simulink model "Joystick_HIL"  (R2025b)
settings: Solver=FixedStepDiscrete  StartTime=0.0  StopTime=inf  RelTol=1e-3
undefined symbols (not defined in the file): battery_voltage, force_table, pwm_list, voltage_list
libraries: ros2lib x3
settings Model: Creator=vulcangrip  LastModifiedBy=vulcangrip
settings OptimizationCC: DefaultParameterBehavior=Inlined  EnhancedBackFolding=on  PassReuseOutputArgsAs=Individual arguments  ZeroExternalMemoryAtStartup=off  ZeroInternalMemoryAtStartup=off  OptimizeBlockOrder=speed  DifferentSizesBufferReuse=on  OptimizationCustomize=off  EfficientTunableParamExpr=on
settings DebuggingCC: ParameterTunabilityLossMsg=error
settings SFSimCC: MATLABDynamicMemAlloc=off  SimTargetLang=C++  SimDLTargetLibrary=mkl-dnn
settings RTWCC: SystemTargetFile=ert.tlc  GenCodeOnly=on  TemplateMakefile=ert_default_tmf  Toolchain=CMake  TargetLang=C++  Description=Embedded Coder
settings CodeAppCC: ForceParamTrailComments=on  IgnoreCustomStorageClasses=off  OperatorAnnotations=on  SimulinkDataObjDesc=on  SFDataObjDesc=on  InsertBlockDesc=on
settings ERTTargetCC: RootIOFormat=Structure reference  ERTCustomFileTemplate=example_file_process.tlc  TargetLangStandard=C++11 (ISO)  GenerateSampleERTMain=on  CodeInterfacePackaging=C++ class  SubcomponentCodeInterfacePackaging=C++ class
settings ConfigComp: CovScope=ReferencedModels

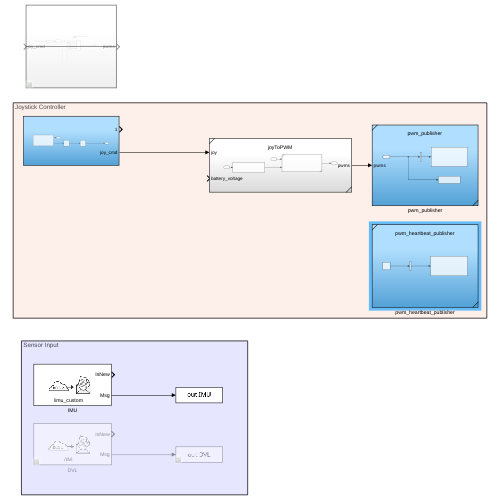
[thumbnail: Simulink's stored preview of the top-level diagram]
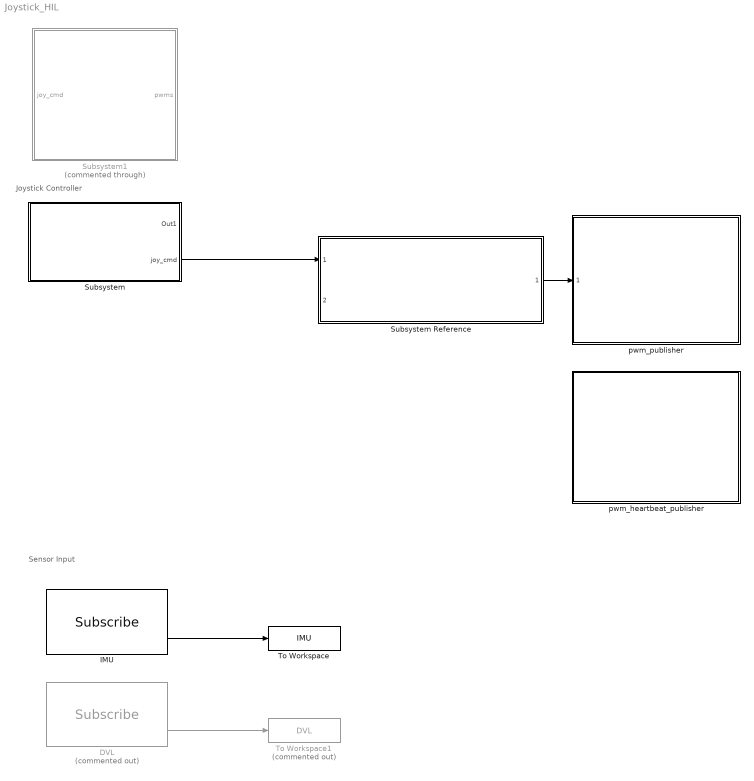
== system Joystick_HIL ==
  note: Joystick Controller
  note: Sensor Input
  DVL : ros2lib/Subscribe  Commented=on  topicSource=Specify your own  topic=/dvl  messageType=custom_interfaces/Position  sampleTime=-1  QOSHistory=Keep last  QOSDepth=10  QOSReliability=Reliable  QOSDurability=Volatile  QOSDeadline=Inf  QOSLifespan=Inf  QOSLiveliness=Automatic  QOSLeaseDuration=Inf  QOSAvoidROSNamespaceConventions=off
  IMU : ros2lib/Subscribe  topicSource=Specify your own  topic=/imu_custom  messageType=custom_interfaces/Imu  sampleTime=-1  QOSHistory=Keep last  QOSDepth=10  QOSReliability=Reliable  QOSDurability=Volatile  QOSDeadline=Inf  QOSLifespan=Inf  QOSLiveliness=Automatic  QOSLeaseDuration=Inf  QOSAvoidROSNamespaceConventions=off
  Subsystem : Subsystem
  Subsystem Reference : Subsystem  ReferencedSubsystem=joyToPWM
  Subsystem1 : Subsystem  Commented=through  TreatAsAtomicUnit=on
  To Workspace : ToWorkspace  VariableName=IMU  SaveFormat=Timeseries  SampleTime=-1
  To Workspace1 : ToWorkspace  Commented=on  VariableName=DVL  SaveFormat=Timeseries  SampleTime=-1
  pwm_heartbeat_publisher : Subsystem  ReferencedSubsystem=pwm_heartbeat_publisher
  pwm_publisher : Subsystem  ReferencedSubsystem=pwm_publisher
  wires:
  Subsystem Reference/1 -> pwm_publisher/1
  Subsystem/2(joy_cmd) -> Subsystem Reference/1
  IMU/2 -> To Workspace/1
  DVL/2 -> To Workspace1/1

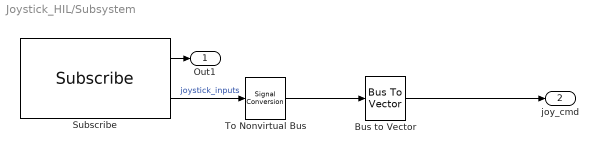
== system Joystick_HIL/Subsystem ==
  Bus to Vector : BusToVector
  Subscribe : ros2lib/Subscribe  topicSource=Specify your own  topic=/ps5_controller  messageType=remote_control_interface/Gamepad  sampleTime=1/60  QOSHistory=Keep last  QOSDepth=10  QOSReliability=Reliable  QOSDurability=Volatile  QOSDeadline=Inf  QOSLifespan=Inf  QOSLiveliness=Automatic  QOSLeaseDuration=Inf  QOSAvoidROSNamespaceConventions=off
  To Nonvirtual Bus : SignalConversion  ConversionOutput=Virtual bus  OverrideOpt=off
  Out1 : Outport
  joy_cmd : Outport  Port=2
  wires:
  To Nonvirtual Bus/1 -> Bus to Vector/1
  Subscribe/2 -> To Nonvirtual Bus/1  "joystick_inputs"
  Subscribe/1 -> Out1/1
  Bus to Vector/1 -> joy_cmd/1

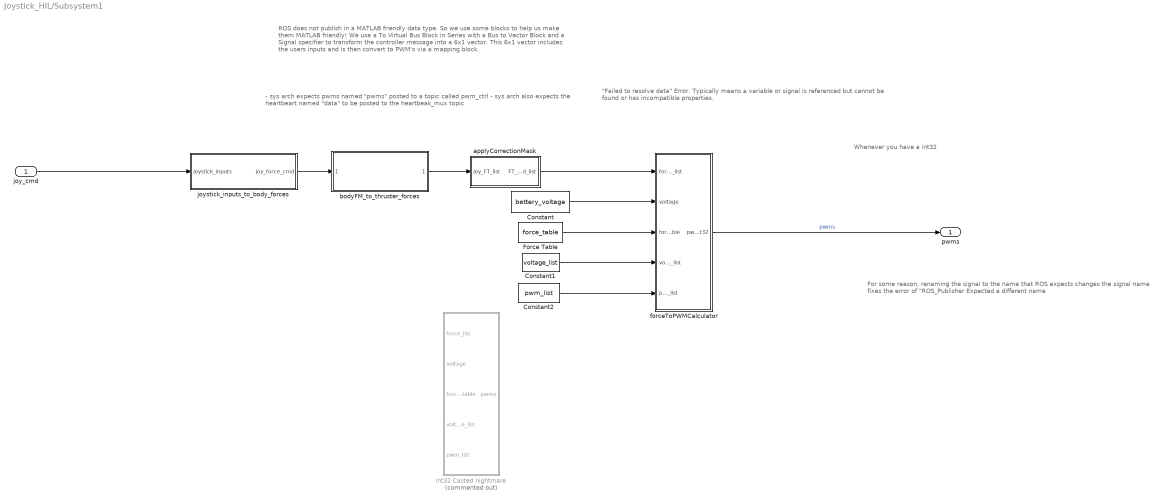
== system Joystick_HIL/Subsystem1 ==
  note: Whenever you have a int32
  note: For some reason, renaming the signal to the name that ROS expects changes the signal name fixes the error of "ROS_Publisher Expected a different name
  note: "Failed to resolve data" Error.
      |
      | Typically means a variable or signal is referenced but cannot be found or has incompatible properties.
  note: ROS does not publish in a MATLAB friendly data type. So we use some blocks to help us make them MATLAB friendly!
      |
      | We use a To Virtual Bus Block in Series with a Bus to Vector Block and a Signal specifier to transform the controller message into a 6x1 vector. This 6x1 vector includes the users inputs and is then convert to PWM's via a mapping block.
  note: - sys arch expects pwms named "pwms" posted to a topic called pwm_ctrl
      | - sys arch also expects the heartbeart  named "data" to be posted to the heartbeak_mux topic
  joy_cmd : Inport
  Constant : Constant  Value=battery_voltage
  Constant1 : Constant  Value=voltage_list
  Constant2 : Constant  Value=pwm_list
  Force Table : Constant  Value=force_table
  applyCorrectionMask : Subsystem
  bodyFM_to_thruster_forces : Subsystem  ReferencedSubsystem=bodyFM_to_thruster_forces
  forceToPWMCalculator : MATLAB Function  TreatAsAtomicUnit=on
  int32 Casted nightmare : MATLAB Function  Commented=on  TreatAsAtomicUnit=on
  joystick_inputs_to_body_forces : MATLAB Function  TreatAsAtomicUnit=on
  pwms : Outport
  wires:
  joystick_inputs_to_body_forces/1(joy_force_cmd) -> bodyFM_to_thruster_forces/1
  bodyFM_to_thruster_forces/1 -> applyCorrectionMask/1(joy_FT_list)
  forceToPWMCalculator/1(pwms_int32) -> pwms/1  "pwms"
  applyCorrectionMask/1(FT_cmd_list) -> forceToPWMCalculator/1(force_list)
  Constant/1 -> forceToPWMCalculator/2(voltage)
  Force Table/1 -> forceToPWMCalculator/3(force_table)
  Constant1/1 -> forceToPWMCalculator/4(voltage_list)
  Constant2/1 -> forceToPWMCalculator/5(pwm_list)
  joy_cmd/1 -> joystick_inputs_to_body_forces/1(joystick_inputs)

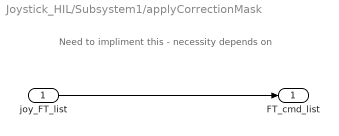
== system Joystick_HIL/Subsystem1/applyCorrectionMask ==
  note: Need to impliment this - necessity depends on
  joy_FT_list : Inport
  FT_cmd_list : Outport
  wires:
  joy_FT_list/1 -> FT_cmd_list/1

== matlab function Joystick_HIL/Subsystem1/forceToPWMCalculator ==
  data: force_list input; pwms_int32 output; voltage input; force_table input; voltage_list input; pwm_list input
function pwms_int32 = forceToPWMCalculator(force_list,voltage,force_table,voltage_list,pwm_list)
%{
This function figures out what pwm to send in order to get the appropriate
force at the current voltage.


%}
pwms = zeros(size(force_list));

for k = 1:length(force_list)
    force = double(force_list(k));

    if(abs(force)<1e-3)
        %if the force setting is very low, just set thruster to stop
        %condition
        pwm_cmd = 1500;
    else
        
        %find the closest voltage less than the input voltage
        [~,closest_index] = min(abs(voltage_list-voltage));
       
        %see if the closest_voltage is above or below the input voltage
        if(closest_index==1)
            %no need to do any interpolation, just take the first column for forces
            lower_voltage_index = 1;
            upper_voltage_index = 1;
    
        elseif(closest_index==length(voltage_list))
            %no need to do any interpolation, just take the last column for forces
            lower_voltage_index = length(voltage_list);
            upper_voltage_index = length(voltage_list);
        elseif(voltage_list(closest_index) < voltage)
            lower_voltage_index = closest_index;
            upper_voltage_index = closest_index+1;
        else
            upper_voltage_index = closest_index;
            lower_voltage_index = closest_index-1;
        end
        
        %average the force column between the two indices\
        if(upper_voltage_index == lower_voltage_index)
            force_column = force_table(lower_voltage_index);
        else
            force_column = force_table(:,lower_voltage_index) + (voltage-voltage_list(lower_voltage_index))*(force_table(:,upper_voltage_index)-force_table(:,lower_voltage_index))/(voltage_list(upper_voltage_index)-voltage_list(lower_voltage_index));
        end
    
        %find the force closest to the input force
        [~,closest_index] = min(abs(force_column-force));
        
        %see if the closest_force is above or below the input force
        if(closest_index==1)
            %no need to do any interpolation, just take the first column for forces
            lower_force_index = 1;
            upper_force_index = 1;
        elseif(closest_index==length(force_list))
            %no need to do any interpolation, just take the last column for forces
            lower_force_index = length(force_list);
            upper_force_index = length(force_list);
        elseif(force_column(closest_index) < force)
            lower_force_index = closest_index;
            upper_force_index = closest_index+1;
        else
            upper_force_index = closest_index;
            lower_force_index = closest_index-1;
        end
        
        %compute scaling coefficient between neighboring forces
        if(lower_force_index == upper_force_index)
            alpha = 0;
        else
            alpha = (force - force_column(upper_force_index))/(force_column(upper_force_index)-force_column(lower_force_index));
        end
    
        %find closest pwm to this force
        pwm_cmd = pwm_list(lower_force_index) + alpha*(pwm_list(upper_force_index)-pwm_list(lower_force_index));
        pwm_cmd = round(pwm_cmd); %round to the nearest integer
    end
    pwms(k) = pwm_cmd;

    pwms_int32 = int32(pwms);
end

== matlab function Joystick_HIL/Subsystem1/int32 Casted nightmare ==
  data: force_list input; voltage input; pwms output; force_table input; voltage_list input; pwm_list input
function pwms = forceToPWMCalculator(force_list,voltage,force_table,voltage_list,pwm_list)

%pwms = int32(force_list*battery_voltage);
%{
This function figures out what pwm to send in order to get the appropriate
force at the current voltage.


%}
pwms = int32(zeros(size(force_list)));

for k = 1:length(force_list)
    force = force_list(k);

    if(abs(force)<1e-3)
        %if the force setting is very low, just set thruster to stop
        %condition
        pwm_cmd = int32(1500);
    else
        
        %find the closest voltage less than the input voltage
        [~,closest_index] = min(abs(voltage_list-voltage));
       
        %see if the closest_voltage is above or below the input voltage
        if(closest_index==int32(1))
            %no need to do any interpolation, just take the first column for forces
            lower_voltage_index = 1;
            upper_voltage_index = 1;
    
        elseif(closest_index==length(voltage_list))
            %no need to do any interpolation, just take the last column for forces
            lower_voltage_index = int32(length(voltage_list));
            upper_voltage_index = int32(length(voltage_list));
        elseif(voltage_list(closest_index) < voltage)
            lower_voltage_index = int32(closest_index);
            upper_voltage_index = int32(closest_index+1);
        else
            upper_voltage_index = int32(closest_index);
            lower_voltage_index = int32(closest_index-1);
        end
        
        %average the force column between the two indices\
        if(upper_voltage_index == lower_voltage_index)
            force_column = force_table(lower_voltage_index);
        else
            force_column = force_table(:,lower_voltage_index) + (voltage-voltage_list(lower_voltage_index))*(force_table(:,upper_voltage_index)-force_table(:,lower_voltage_index))/(voltage_list(upper_voltage_index)-voltage_list(lower_voltage_index));
        end
    
        %find the force closest to the input force
        [~,closest_index] = min(abs(force_column-force));
        
        %see if the closest_force is above or below the input force
        if(closest_index==int32(1))
            %no need to do any interpolation, just take the first column for forces
            lower_force_index = int32(1);
            upper_force_index = int32(1);
        elseif(closest_index==length(force_list))
            %no need to do any interpolation, just take the last column for forces
            lower_force_index = int32(length(force_list));
            upper_force_index = int32(length(force_list));
        elseif(force_column(closest_index) < force)
            lower_force_index = int32(closest_index);
            upper_force_index = int32(closest_index+1);
        else
            upper_force_index = int32(closest_index);
            lower_force_index = int32(closest_index-1);
        end
        
        %compute scaling coefficient between neighboring forces
        if(lower_force_index == upper_force_index)
            alpha = int32(0);
        else
            alpha = (force - force_column(upper_force_index))/(force_column(upper_force_index)-force_column(lower_force_index));
        end
    
        %find closest pwm to this force
        pwm_cmd = pwm_list(lower_force_index) + alpha*(pwm_list(upper_force_index)-pwm_list(lower_force_index));
        pwm_cmd = round(pwm_cmd); %round to the nearest integer
    end
    pwms(k) = pwm_cmd;
end

== matlab function Joystick_HIL/Subsystem1/joystick_inputs_to_body_forces ==
  data: joystick_inputs input; joy_force_cmd output
function joy_force_cmd = fcn(joystick_inputs)

%Create the mapping here for PWM values.
%Recall that PWM 1-8 correspond to thruster postions which follow,

%pwm of each thruster on the robot
%In left to right:
%f = front / r = rear
%l = left  / r = right
%t = top   / b = bottom
%PWM(1)=pwm_flt
%PWM(2)=pwm_frt
%PWM(3)=pwm_rlt
%PWM(4)=pwm_rrt
%PWM(5)=pwm_flb
%PWM(6)=pwm_frb
%PWM(7)=pwm_rlb
%PWM(8)=pwm_rrb

%unpacking joystick inputs
x = joystick_inputs(1);
y = joystick_inputs(2);
pitch = joystick_inputs(3);
yaw = joystick_inputs(4);
sink = joystick_inputs(5);
rise = joystick_inputs(6);

joy_force_cmd = joystick_inputs;

%Need to specify int32 for the output data type to maintain consistent
